simulink model "testModel"  (R2024b)
settings: Solver=ode8  StartTime=0.0  StopTime=10.0  FixedStep=0.025  RelTol=1e-3
values from neighbouring files (symbols this model uses):
  I = diag(Iv)    [InitTest.m]
  invI = inv(I)    [InitTest.m]
  R = 42000000    [InitTest.m]
  w0 = [1e-6; 1e-6; orb.n]    [InitTest.m]
undefined symbols (not defined in the file or in its folder): env, flag, IC, orb
libraries: matrix_library x2
settings Model: SimulationMode=accelerator  Creator=elisa  LastModifiedBy=filippocamaleonte

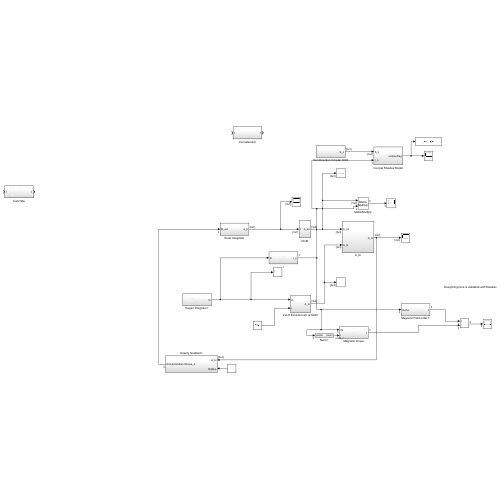
[thumbnail: Simulink's stored preview of the top-level diagram]
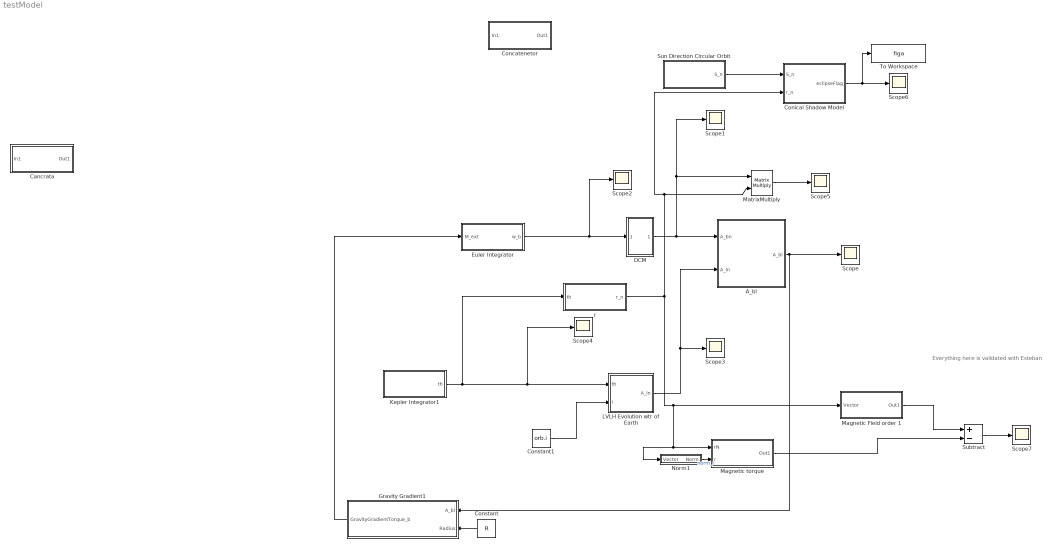
== system testModel ==
  note: Everything here is validated with Esteban
  A_bl : Subsystem
  Cancrata : Subsystem
  Concatenetor : Subsystem
  Conical Shadow Model : Subsystem
  Constant : Constant  Value=R
  Constant1 : Constant  Value=orb.i
  DCM : Subsystem
  Euler Integrator : Subsystem
  Gravity Gradient1 : Subsystem
  Kepler Integrator1 : Subsystem
  LVLH Evolution wtr of Earth : Subsystem
  Magnetic Field order 1 : Subsystem
  Magnetic torque : Subsystem
  MatrixMultiply : Product  Multiplication=Matrix(*)
  Norm1 : Subsystem
  Scope{,1..7} (8 alike) : Scope
  Subtract : Sum  Inputs=+-
  Sun Direction Circular Orbit : Subsystem
  To Workspace : ToWorkspace  VariableName=figa  SampleTime=-1
  r : Subsystem
  wires:
  Euler Integrator/1(w_b) -> Scope2/1, DCM/1(In1)
  DCM/1(A_bn) -> Scope1/1, MatrixMultiply/1, A_bl/1(A_bn)
  LVLH Evolution wtr of Earth/1(A_ln) -> Scope3/1, A_bl/2(A_ln)
  A_bl/1(A_bl) -> Scope/1, Gravity Gradient1/1(A_bl)
  Constant/1 -> Gravity Gradient1/2(Radius)
  Gravity Gradient1/1(GravityGradientTorque_b) -> Euler Integrator/1(M_ext)
  Kepler Integrator1/1(th) -> r/1(th), LVLH Evolution wtr of Earth/1(th), Scope4/1
  Constant1/1 -> LVLH Evolution wtr of Earth/2(i)
  MatrixMultiply/1 -> Scope5/1
  Sun Direction Circular Orbit/1(S_n) -> Conical Shadow Model/1(S_n)
  Conical Shadow Model/1(eclipseFlag) -> To Workspace/1, Scope6/1
  Norm1/1(Norm) -> Magnetic torque/2(r)  "norm_r"
  r/1(r_n) -> Norm1/1(Vector), Magnetic torque/1(rN), Magnetic Field order 1/1(Vector), MatrixMultiply/2, Conical Shadow Model/2(r_n)
  Subtract/1 -> Scope7/1
  Magnetic Field order 1/1(Out1) -> Subtract/1
  Magnetic torque/1(Out1) -> Subtract/2

== system testModel/A_bl ==
  A_bn : Inport
  A_ln : Inport  Port=2
  Matrix Multiply : Product  Multiplication=Matrix(*)
  Transpose : Math  Operator=transpose
  A_bl : Outport
  wires:
  Transpose/1 -> Matrix Multiply/2
  A_ln/1 -> Transpose/1
  Matrix Multiply/1 -> A_bl/1
  A_bn/1 -> Matrix Multiply/1

== system testModel/Cancrata ==
  In1 : Inport
  K_nm : Subsystem
  P_0 : Subsystem
  Pnn : Subsystem
  dPnn : Subsystem
  Out1 : Outport
  wires:
  In1/1 -> Out1/1

== system testModel/Concatenetor ==
  In1 : Inport
  Matrix Concatenate : Concatenate  NumInputs=3  Mode=Multidimensional array  ConcatenateDimension=2
  Out1 : Outport
  wires:
  Matrix Concatenate/1 -> Out1/1
  In1/1 -> Matrix Concatenate/3, Matrix Concatenate/1, Matrix Concatenate/2

== system testModel/Conical Shadow Model ==
  note: Output Interface
  note: Input Interface
  note: Model is cylindrical shadow, formula was taken by Crassidis
  S_n : Inport
  r_n : Inport  Port=2
  Dot Product : DotProduct  OutDataTypeStr=Inherit: Inherit via internal rule
  Earth's Radius : Constant  Value=env.Earth.R
  Eclipse (1) : Subsystem  TreatAsAtomicUnit=on
  Gain : Gain  Gain=-1
  If : If  NumInputs=2  IfExpression=u1 < u2
  Merge : Merge
  Norm : Subsystem
  NotEclipse (0) : Subsystem  TreatAsAtomicUnit=on
  Sqrt : Sqrt
  Square : Math  Operator=square
  Square1 : Math  Operator=square
  Subtract : Sum  Inputs=+-
  eclipseFlag : Outport
  wires:
  r_n/1 -> Dot Product/2, Norm/1(Vector)  "r_n"
  S_n/1 -> Dot Product/1  "S_n"
  Norm/1(Norm) -> Square1/1  "norm_r"
  If/1 -> Eclipse (1)/Action
  If/2 -> NotEclipse (0)/Action
  Merge/1 -> eclipseFlag/1
  Eclipse (1)/1(One) -> Merge/1
  NotEclipse (0)/1(Zero) -> Merge/2
  Dot Product/1 -> If/1
  Gain/1 -> If/2
  Sqrt/1 -> Gain/1
  Subtract/1 -> Sqrt/1
  Square/1 -> Subtract/2
  Square1/1 -> Subtract/1
  Earth's Radius/1 -> Square/1  "earth_R"

== system testModel/DCM ==
  In1 : Inport
  A312 : Subsystem
  Constant3 : Constant  Value=IC.angles
  Gain : Gain  Gain=-1
  Integrator1 : Integrator  InitialConditionSource=external
  Product1 : Product  Multiplication=Matrix(*)
  Subsystem : Subsystem
  Subsystem1 : Subsystem
  Subsystem2 : Subsystem
  w^ : Subsystem
  A_bn : Outport
  wires:
  w^/1(Out1) -> Gain/1
  Gain/1 -> Product1/1
  In1/1 -> w^/1(In1)
  Product1/1 -> Integrator1/1
  Constant3/1 -> A312/1(In1)
  Integrator1/1 -> Subsystem/1(In1)
  Subsystem/1(Out1) -> Subsystem1/1(In1)
  A312/1(Out1) -> Integrator1/2
  Subsystem1/1(Out1) -> Subsystem2/1(In1)
  Subsystem2/1(Out1) -> Product1/2, A_bn/1

== system testModel/Euler Integrator ==
  M_ext : Inport
  Constant : Constant  Value=I
  Constant1 : Constant  Value=w0  VectorParams1D=off
  Constant2 : Constant  Value=invI
  Cross Product : matrix_library/Cross Product
  Divide : Product  Inputs=**  Multiplication=Matrix(*)
  Integrator : Integrator  InitialConditionSource=external
  Product : Product  Multiplication=Matrix(*)
  Sum : Sum  Inputs=|++
  w_b : Outport
  wires:
  Product/1 -> Cross Product/1
  Divide/1 -> Integrator/1
  Constant/1 -> Product/1
  Constant2/1 -> Divide/1
  Integrator/1 -> Product/2, Cross Product/2, w_b/1
  Constant1/1 -> Integrator/2
  Cross Product/1 -> Sum/1
  Sum/1 -> Divide/2
  M_ext/1 -> Sum/2

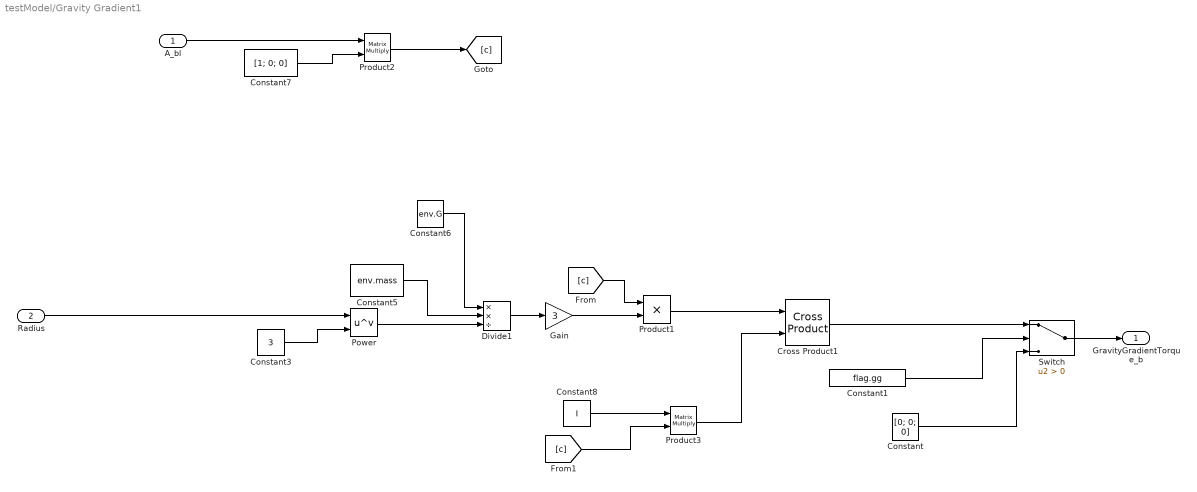
== system testModel/Gravity Gradient1 ==
  A_bl : Inport
  Radius : Inport  Port=2
  Constant : Constant  Value=[0; 0; 0]
  Constant1 : Constant  Value=flag.gg
  Constant3 : Constant  Value=3
  Constant5 : Constant  Value=env.mass
  Constant6 : Constant  Value=env.G
  Constant7 : Constant  Value=[1; 0; 0]
  Constant8 : Constant  Value=I
  Cross Product1 : matrix_library/Cross Product
  Divide1 : Product  Inputs=**/
  Gain : Gain  Gain=3
  Power : Math  Operator=pow
  Product1 : Product
  Product2 : Product  Multiplication=Matrix(*)
  Product3 : Product  Multiplication=Matrix(*)
  Switch : Switch  Criteria=u2 > Threshold  SaturateOnIntegerOverflow=off  InputSameDT=off
  GravityGradientTorque_b : Outport
  wires:
  A_bl/1 -> Product2/1
  Product3/1 -> Cross Product1/2
  Product2/1 -> [c]
  Constant8/1 -> Product3/1
  Product1/1 -> Cross Product1/1
  [c] -> Product1/1
  [c] -> Product3/2
  Constant6/1 -> Divide1/1
  Constant5/1 -> Divide1/2
  Radius/1 -> Power/1
  Constant7/1 -> Product2/2
  Constant3/1 -> Power/2
  Power/1 -> Divide1/3
  Divide1/1 -> Gain/1
  Gain/1 -> Product1/2
  Constant/1 -> Switch/3
  Switch/1 -> GravityGradientTorque_b/1
  Cross Product1/1 -> Switch/1
  Constant1/1 -> Switch/2

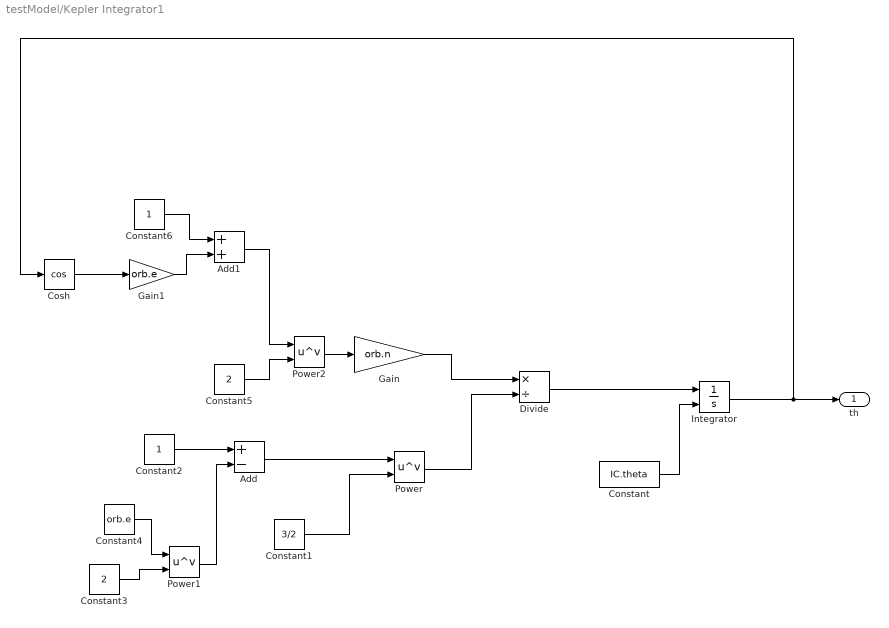
== system testModel/Kepler Integrator1 ==
  Add : Sum  Inputs=+-
  Add1 : Sum
  Constant : Constant  Value=IC.theta
  Constant1 : Constant  Value=3/2
  Constant2 : Constant
  Constant3 : Constant  Value=2
  Constant4 : Constant  Value=orb.e
  Constant5 : Constant  Value=2
  Constant6 : Constant
  Cosh : Trigonometry  Operator=cos
  Divide : Product  Inputs=*/
  Gain : Gain  Gain=orb.n
  Gain1 : Gain  Gain=orb.e
  Integrator : Integrator  InitialConditionSource=external  WrapState=on  WrappedStateUpperValue=2*pi  WrappedStateLowerValue=0
  Power : Math  Operator=pow
  Power1 : Math  Operator=pow
  Power2 : Math  Operator=pow
  th : Outport
  wires:
  Constant/1 -> Integrator/2
  Integrator/1 -> Cosh/1, th/1
  Divide/1 -> Integrator/1
  Power/1 -> Divide/2
  Constant1/1 -> Power/2
  Constant2/1 -> Add/1
  Add/1 -> Power/1
  Power1/1 -> Add/2
  Constant3/1 -> Power1/2
  Constant4/1 -> Power1/1
  Gain/1 -> Divide/1
  Power2/1 -> Gain/1
  Constant5/1 -> Power2/2
  Add1/1 -> Power2/1
  Constant6/1 -> Add1/1
  Gain1/1 -> Add1/2
  Cosh/1 -> Gain1/1

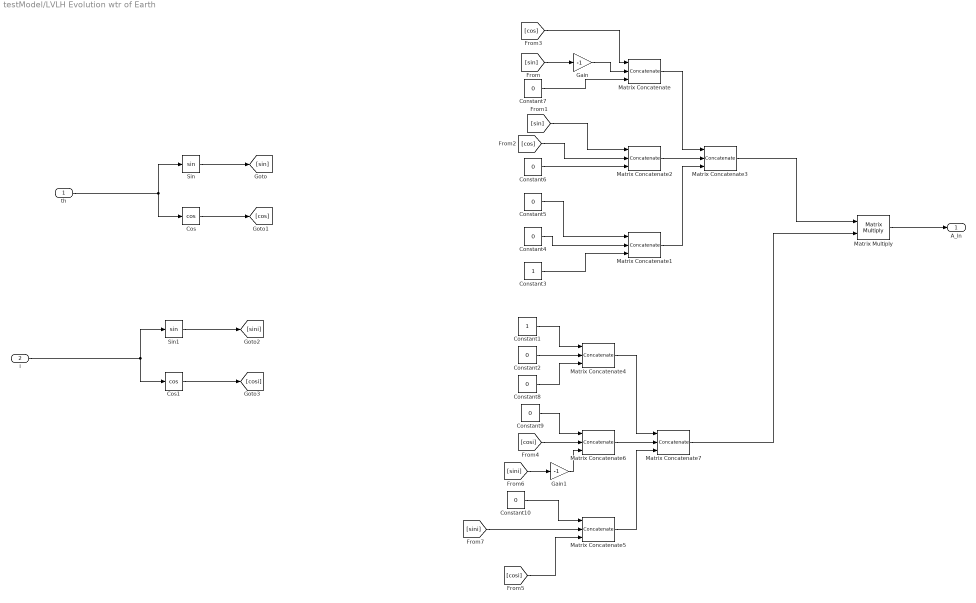
== system testModel/LVLH Evolution wtr of Earth ==
  th : Inport
  i : Inport  Port=2
  Constant1 : Constant
  Constant{2,4..10} (8 alike) : Constant  Value=0
  Constant3 : Constant
  Cos : Trigonometry  Operator=cos
  Cos1 : Trigonometry  Operator=cos
  Gain : Gain  Gain=-1
  Gain1 : Gain  Gain=-1
  Matrix Concatenate{,1..2,4..6} (6 alike) : Concatenate  NumInputs=3  Mode=Multidimensional array
  Matrix Concatenate3 : Concatenate  NumInputs=3  Mode=Multidimensional array  ConcatenateDimension=2
  Matrix Concatenate7 : Concatenate  NumInputs=3  Mode=Multidimensional array  ConcatenateDimension=2
  Matrix Multiply : Product  Multiplication=Matrix(*)
  Sin : Trigonometry
  Sin1 : Trigonometry
  A_ln : Outport
  wires:
  Cos/1 -> [cos]
  Matrix Concatenate1/1 -> Matrix Concatenate3/3
  th/1 -> Cos/1, Sin/1
  Matrix Concatenate/1 -> Matrix Concatenate3/1
  Constant5/1 -> Matrix Concatenate1/1
  Constant3/1 -> Matrix Concatenate1/3
  [cos] -> Matrix Concatenate/1
  Sin/1 -> [sin]
  Constant6/1 -> Matrix Concatenate2/3
  Constant7/1 -> Matrix Concatenate/3
  Constant4/1 -> Matrix Concatenate1/2
  Matrix Concatenate2/1 -> Matrix Concatenate3/2
  [cos] -> Matrix Concatenate2/2
  [sin] -> Matrix Concatenate2/1
  Gain/1 -> Matrix Concatenate/2
  [sin] -> Gain/1
  Cos1/1 -> [cosi]
  Sin1/1 -> [sini]
  i/1 -> Cos1/1, Sin1/1
  Matrix Multiply/1 -> A_ln/1
  Matrix Concatenate3/1 -> Matrix Multiply/1
  Matrix Concatenate7/1 -> Matrix Multiply/2
  Matrix Concatenate6/1 -> Matrix Concatenate7/2
  Matrix Concatenate5/1 -> Matrix Concatenate7/3
  Matrix Concatenate4/1 -> Matrix Concatenate7/1
  Constant1/1 -> Matrix Concatenate4/1
  Constant2/1 -> Matrix Concatenate4/2
  Constant8/1 -> Matrix Concatenate4/3
  Constant9/1 -> Matrix Concatenate6/1
  Constant10/1 -> Matrix Concatenate5/1
  [cosi] -> Matrix Concatenate5/3
  [cosi] -> Matrix Concatenate6/2
  [sini] -> Matrix Concatenate5/2
  [sini] -> Gain1/1
  Gain1/1 -> Matrix Concatenate6/3

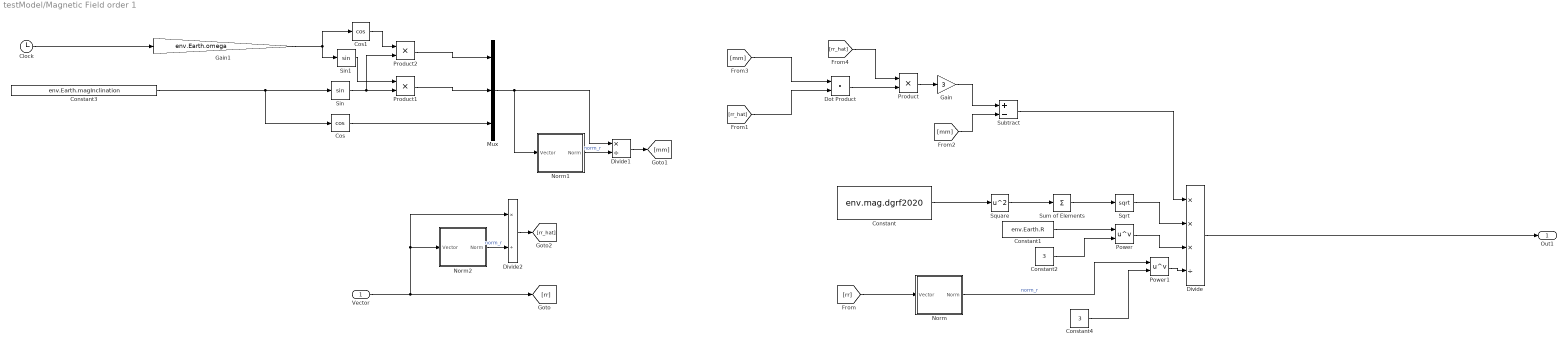
== system testModel/Magnetic Field order 1 ==
  Vector : Inport
  Clock : Clock
  Constant : Constant  Value=env.mag.dgrf2020
  Constant1 : Constant  Value=env.Earth.R
  Constant2 : Constant  Value=3
  Constant3 : Constant  Value=env.Earth.magInclination
  Constant4 : Constant  Value=3
  Cos : Trigonometry  Operator=cos
  Cos1 : Trigonometry  Operator=cos
  Divide : Product  Inputs=***/
  Divide1 : Product  Inputs=*/
  Divide2 : Product  Inputs=*/
  Dot Product : DotProduct  OutDataTypeStr=Inherit: Inherit via internal rule
  Gain : Gain  Gain=3
  Gain1 : Gain  Gain=env.Earth.omega
  Mux : Mux  Inputs=3
  Norm : Subsystem
  Norm1 : Subsystem
  Norm2 : Subsystem
  Power : Math  Operator=pow
  Power1 : Math  Operator=pow
  Product : Product
  Product1 : Product
  Product2 : Product
  Sin : Trigonometry
  Sin1 : Trigonometry
  Sqrt : Sqrt
  Square : Math  Operator=square
  Subtract : Sum  Inputs=+-
  Sum of Elements : Sum  Inputs=+
  Out1 : Outport
  wires:
  Constant/1 -> Square/1
  Square/1 -> Sum of Elements/1
  Sum of Elements/1 -> Sqrt/1
  Constant1/1 -> Power/1
  Constant2/1 -> Power/2
  Sqrt/1 -> Divide/2
  Power/1 -> Divide/3
  Constant4/1 -> Power1/2
  Power1/1 -> Divide/4
  Norm/1(Norm) -> Power1/1  "norm_r"
  Vector/1 -> Norm2/1(Vector), Divide2/1, [rr]
  [rr] -> Norm/1(Vector)
  [rr_hat] -> Dot Product/2
  Subtract/1 -> Divide/1
  [mm] -> Subtract/2
  Dot Product/1 -> Product/2
  Product/1 -> Gain/1
  Gain/1 -> Subtract/1
  [rr_hat] -> Product/1
  [mm] -> Dot Product/1
  Mux/1 -> Norm1/1(Vector), Divide1/1
  Cos/1 -> Mux/3
  Constant3/1 -> Sin/1, Cos/1
  Clock/1 -> Gain1/1
  Sin/1 -> Product2/2, Product1/2
  Product1/1 -> Mux/2
  Product2/1 -> Mux/1
  Cos1/1 -> Product2/1
  Gain1/1 -> Cos1/1, Sin1/1
  Sin1/1 -> Product1/1
  Divide/1 -> Out1/1
  Norm1/1(Norm) -> Divide1/2  "norm_r"
  Divide1/1 -> [mm]
  Norm2/1(Norm) -> Divide2/2  "norm_r"
  Divide2/1 -> [rr_hat]

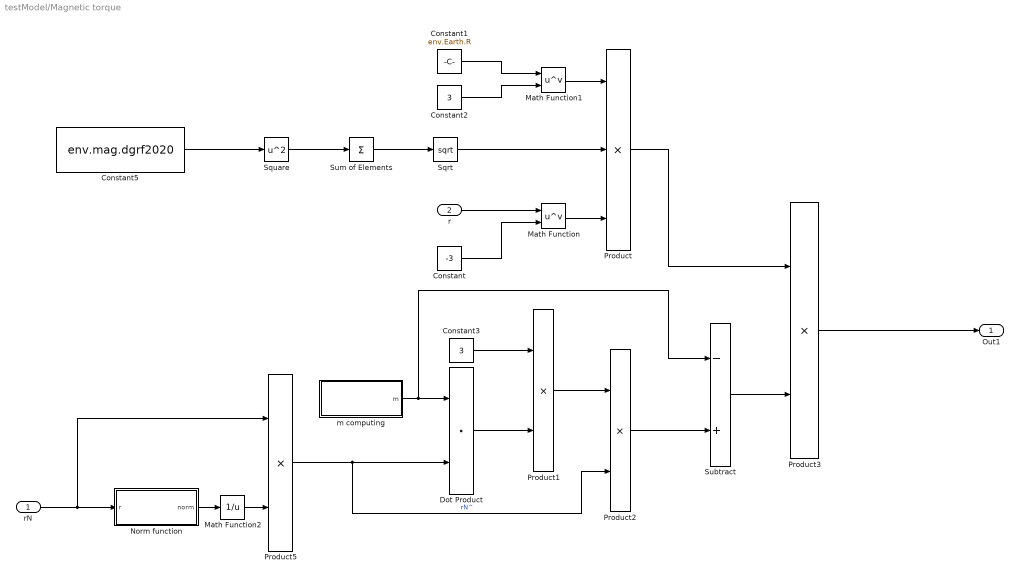
== system testModel/Magnetic torque ==
  rN : Inport
  r : Inport  Port=2
  Constant : Constant  Value=-3
  Constant1 : Constant  Value=env.Earth.R
  Constant2 : Constant  Value=3
  Constant3 : Constant  Value=3
  Constant5 : Constant  Value=env.mag.dgrf2020
  Dot Product : DotProduct  OutDataTypeStr=Inherit: Inherit via internal rule
  Math Function : Math  Operator=pow
  Math Function1 : Math  Operator=pow
  Math Function2 : Math  Operator=reciprocal
  Norm function : Subsystem
  Product : Product  Inputs=3
  Product{1..3,5} (4 alike) : Product
  Sqrt : Sqrt
  Square : Math  Operator=square
  Subtract : Sum  Inputs=-+
  Sum of Elements : Sum  Inputs=+
  m computing : Subsystem
  Out1 : Outport
  wires:
  Sqrt/1 -> Product/2
  Constant3/1 -> Product1/1
  Math Function1/1 -> Product/1
  Product/1 -> Product3/1
  Product1/1 -> Product2/1
  Math Function2/1 -> Product5/2
  Constant/1 -> Math Function/2
  Dot Product/1 -> Product1/2
  Product5/1 -> Dot Product/2, Product2/2  "rN^"
  Constant1/1 -> Math Function1/1
  Constant2/1 -> Math Function1/2
  Product2/1 -> Subtract/2
  rN/1 -> Product5/1, Norm function/1(r)
  Norm function/1(norm) -> Math Function2/1
  r/1 -> Math Function/1
  m computing/1(m) -> Dot Product/1, Subtract/1
  Math Function/1 -> Product/3
  Subtract/1 -> Product3/2
  Sum of Elements/1 -> Sqrt/1
  Constant5/1 -> Square/1
  Square/1 -> Sum of Elements/1
  Product3/1 -> Out1/1

== system testModel/Norm1 ==
  Vector : Inport
  Add : Sum  Inputs=+++
  Demux : Demux  Outputs=3
  Sqrt : Sqrt
  Square : Math  Operator=square
  Square1 : Math  Operator=square
  Square2 : Math  Operator=square
  Norm : Outport
  wires:
  Square/1 -> Add/1
  Add/1 -> Sqrt/1
  Demux/3 -> Square1/1
  Square2/1 -> Add/2
  Square1/1 -> Add/3
  Demux/1 -> Square/1
  Demux/2 -> Square2/1
  Vector/1 -> Demux/1
  Sqrt/1 -> Norm/1

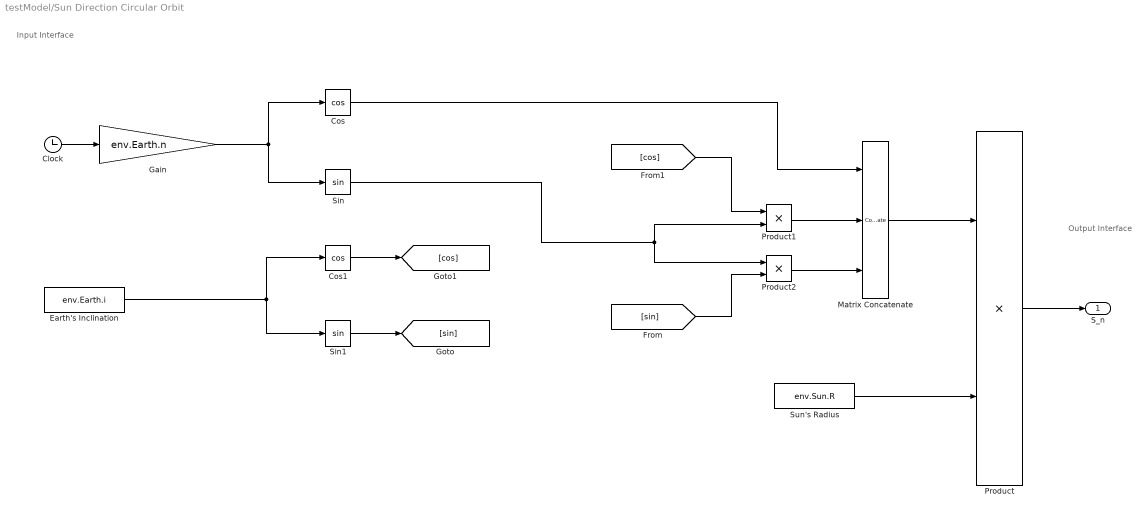
== system testModel/Sun Direction Circular Orbit ==
  note: Input Interface
  note: Output Interface
  Clock : Clock
  Cos : Trigonometry  Operator=cos
  Cos1 : Trigonometry  Operator=cos
  Earth's Inclination : Constant  Value=env.Earth.i
  Gain : Gain  Gain=env.Earth.n
  Matrix Concatenate : Concatenate  NumInputs=3  Mode=Multidimensional array
  Product : Product
  Product1 : Product
  Product2 : Product
  Sin : Trigonometry
  Sin1 : Trigonometry
  Sun's Radius : Constant  Value=env.Sun.R
  S_n : Outport
  wires:
  Clock/1 -> Gain/1
  Gain/1 -> Sin/1, Cos/1
  Product/1 -> S_n/1
  Sun's Radius/1 -> Product/2
  Matrix Concatenate/1 -> Product/1
  Earth's Inclination/1 -> Sin1/1, Cos1/1
  Cos1/1 -> [cos]
  Sin1/1 -> [sin]
  Cos/1 -> Matrix Concatenate/1
  Product1/1 -> Matrix Concatenate/2
  Product2/1 -> Matrix Concatenate/3
  [sin] -> Product2/2
  [cos] -> Product1/1
  Sin/1 -> Product1/2, Product2/1

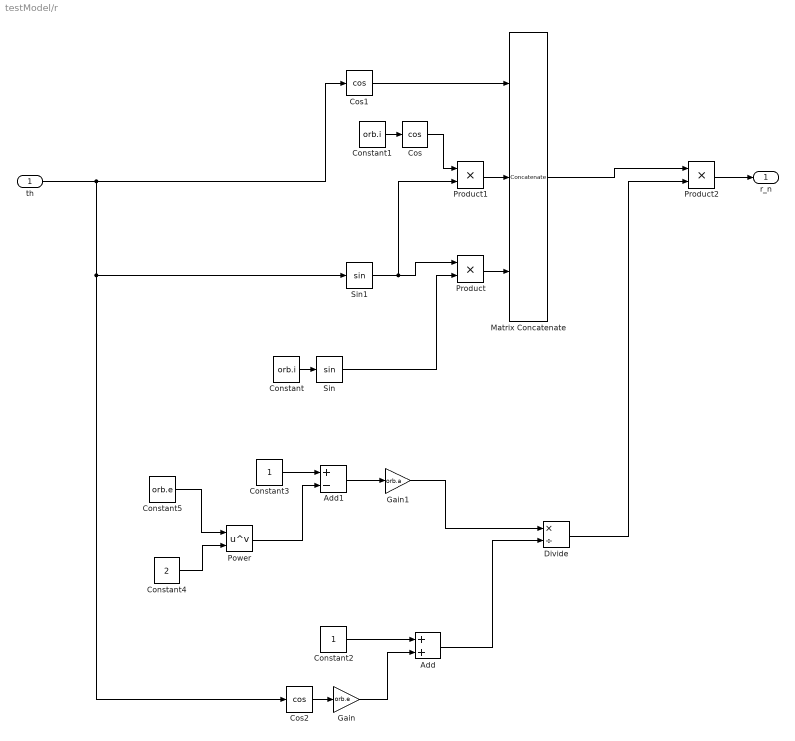
== system testModel/r ==
  th : Inport
  Add : Sum
  Add1 : Sum  Inputs=+-
  Constant : Constant  Value=orb.i
  Constant1 : Constant  Value=orb.i
  Constant2 : Constant
  Constant3 : Constant
  Constant4 : Constant  Value=2
  Constant5 : Constant  Value=orb.e
  Cos : Trigonometry  Operator=cos
  Cos1 : Trigonometry  Operator=cos
  Cos2 : Trigonometry  Operator=cos
  Divide : Product  Inputs=*/
  Gain : Gain  Gain=orb.e
  Gain1 : Gain  Gain=orb.a
  Matrix Concatenate : Concatenate  NumInputs=3  Mode=Multidimensional array
  Power : Math  Operator=pow
  Product : Product
  Product1 : Product
  Product2 : Product
  Sin : Trigonometry
  Sin1 : Trigonometry
  r_n : Outport
  wires:
  Constant/1 -> Sin/1
  Cos1/1 -> Matrix Concatenate/1
  th/1 -> Sin1/1, Cos2/1, Cos1/1
  Product1/1 -> Matrix Concatenate/2
  Product/1 -> Matrix Concatenate/3
  Sin1/1 -> Product1/2, Product/1
  Sin/1 -> Product/2
  Constant1/1 -> Cos/1
  Cos/1 -> Product1/1
  Product2/1 -> r_n/1
  Matrix Concatenate/1 -> Product2/1
  Divide/1 -> Product2/2
  Constant2/1 -> Add/1
  Add/1 -> Divide/2
  Cos2/1 -> Gain/1
  Gain/1 -> Add/2
  Constant3/1 -> Add1/1
  Power/1 -> Add1/2
  Constant4/1 -> Power/2
  Constant5/1 -> Power/1
  Add1/1 -> Gain1/1
  Gain1/1 -> Divide/1

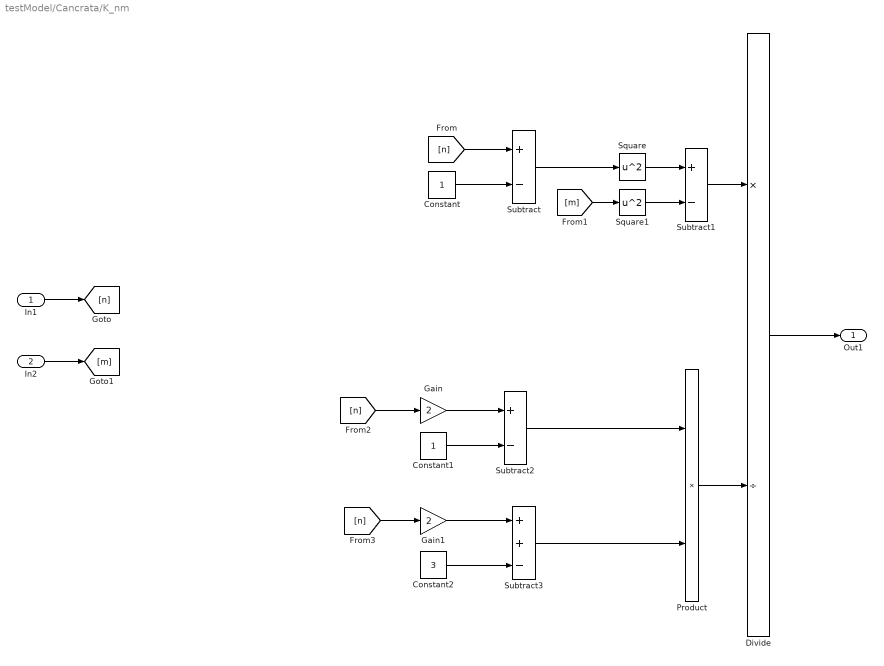
== system testModel/Cancrata/K_nm ==
  In1 : Inport
  In2 : Inport  Port=2
  Constant : Constant
  Constant1 : Constant
  Constant2 : Constant  Value=3
  Divide : Product  Inputs=*/
  Gain : Gain  Gain=2
  Gain1 : Gain  Gain=2
  Product : Product
  Square : Math  Operator=square
  Square1 : Math  Operator=square
  Subtract : Sum  Inputs=+-
  Subtract1 : Sum  Inputs=+-
  Subtract2 : Sum  Inputs=+-
  Subtract3 : Sum  Inputs=++-
  Out1 : Outport
  wires:
  In1/1 -> [n]
  In2/1 -> [m]
  [n] -> Subtract/1
  Constant/1 -> Subtract/2
  Subtract/1 -> Square/1
  Square/1 -> Subtract1/1
  [m] -> Square1/1
  Square1/1 -> Subtract1/2
  Subtract1/1 -> Divide/1
  Divide/1 -> Out1/1
  Product/1 -> Divide/2
  [n] -> Gain/1
  Constant1/1 -> Subtract2/2
  Gain/1 -> Subtract2/1
  Subtract2/1 -> Product/1
  Subtract3/1 -> Product/2
  Constant2/1 -> Subtract3/3
  Gain1/1 -> Subtract3/1
  [n] -> Gain1/1

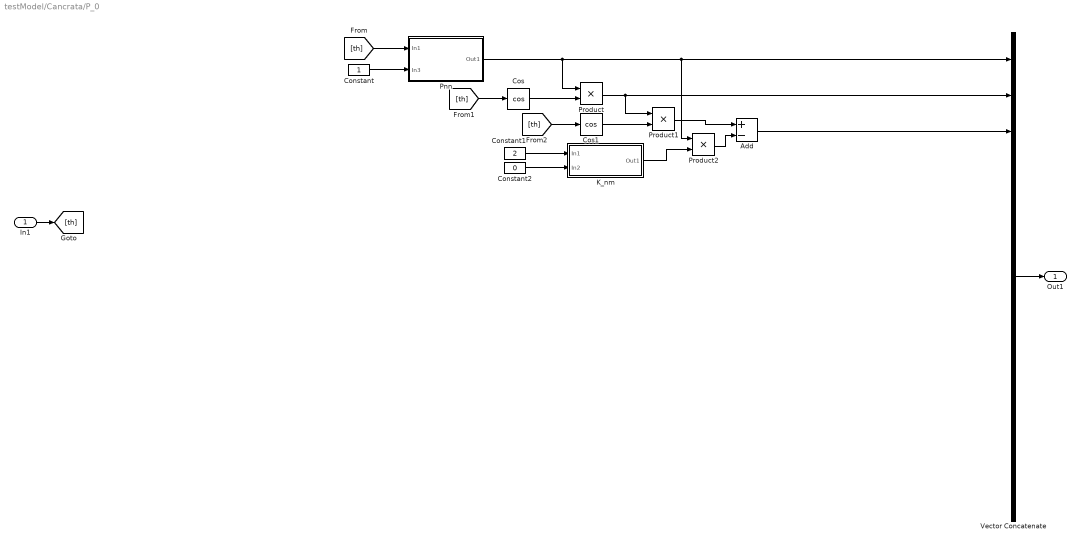
== system testModel/Cancrata/P_0 ==
  In1 : Inport
  Add : Sum  Inputs=+-
  Constant : Constant
  Constant1 : Constant  Value=2
  Constant2 : Constant  Value=0
  Cos : Trigonometry  Operator=cos
  Cos1 : Trigonometry  Operator=cos
  K_nm : Subsystem
  Pnn : Subsystem
  Product : Product
  Product1 : Product
  Product2 : Product
  Vector Concatenate : Concatenate  NumInputs=13
  Out1 : Outport
  wires:
  Vector Concatenate/1 -> Out1/1
  Constant/1 -> Pnn/2(In3)
  In1/1 -> [th]
  [th] -> Pnn/1(In1)
  Pnn/1(Out1) -> Product2/1, Vector Concatenate/1, Product/1
  Constant2/1 -> K_nm/2(In2)
  Constant1/1 -> K_nm/1(In1)
  [th] -> Cos/1
  Cos/1 -> Product/2
  Product/1 -> Product1/1, Vector Concatenate/2
  Cos1/1 -> Product1/2
  [th] -> Cos1/1
  Add/1 -> Vector Concatenate/3
  Product1/1 -> Add/1
  K_nm/1(Out1) -> Product2/2
  Product2/1 -> Add/2

== system testModel/Cancrata/Pnn ==
  In1 : Inport
  In3 : Inport  Port=2
  Power : Math  Operator=pow
  Sin : Trigonometry
  Out1 : Outport
  wires:
  In3/1 -> Sin/1
  In1/1 -> Power/2
  Sin/1 -> Power/1
  Power/1 -> Out1/1

== system testModel/Cancrata/dPnn ==
  In1 : Inport
  In2 : Inport  Port=2
  Constant : Constant
  Cos : Trigonometry  Operator=cos
  Power : Math  Operator=pow
  Product : Product  Inputs=3
  Sin : Trigonometry
  Subtract : Sum  Inputs=+-
  Out1 : Outport
  wires:
  In2/1 -> Cos/1, Sin/1
  Sin/1 -> Power/1
  In1/1 -> Product/3, Subtract/1
  Constant/1 -> Subtract/2
  Subtract/1 -> Power/2
  Product/1 -> Out1/1
  Cos/1 -> Product/1
  Power/1 -> Product/2

== system testModel/Conical Shadow Model/Eclipse (1) ==
  Action Port : ActionPort  ActionPortLabel=if(u1 < u2)
  Constant : Constant
  One : Outport
  wires:
  Constant/1 -> One/1

== system testModel/Conical Shadow Model/Norm ==
  Vector : Inport
  Add : Sum  Inputs=+++
  Demux : Demux  Outputs=3
  Sqrt : Sqrt
  Square : Math  Operator=square
  Square1 : Math  Operator=square
  Square2 : Math  Operator=square
  Norm : Outport
  wires:
  Square/1 -> Add/1
  Add/1 -> Sqrt/1
  Demux/3 -> Square1/1
  Square2/1 -> Add/2
  Square1/1 -> Add/3
  Demux/1 -> Square/1
  Demux/2 -> Square2/1
  Vector/1 -> Demux/1
  Sqrt/1 -> Norm/1

== system testModel/Conical Shadow Model/NotEclipse (0) ==
  Action Port : ActionPort  ActionPortLabel=else
  Constant : Constant  Value=0
  Zero : Outport
  wires:
  Constant/1 -> Zero/1

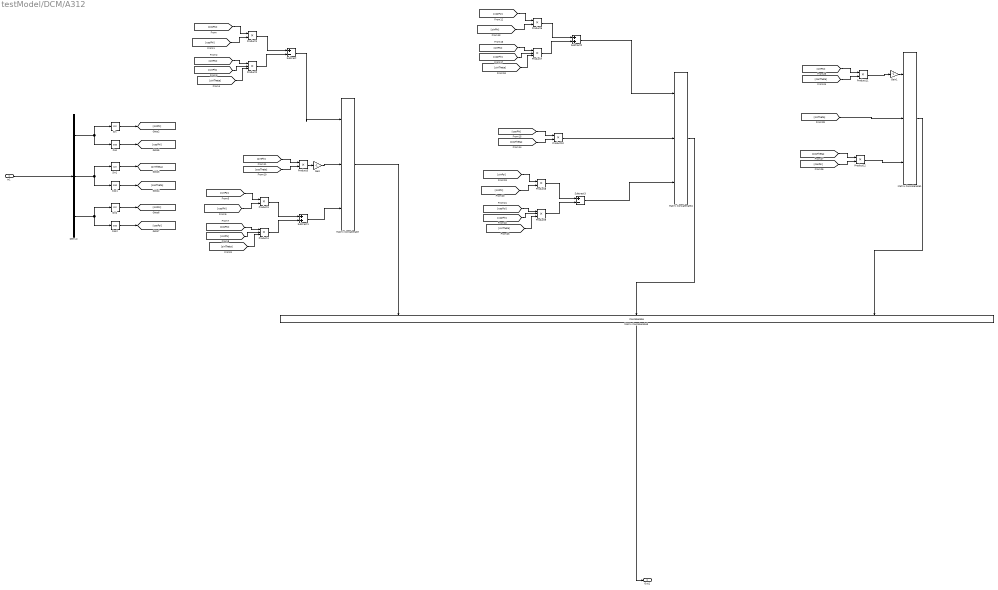
== system testModel/DCM/A312 ==
  In1 : Inport
  Cos : Trigonometry  Operator=cos
  Cos1 : Trigonometry  Operator=cos
  Cos2 : Trigonometry  Operator=cos
  Demux : Demux  Outputs=3
  Gain : Gain  Gain=-1
  Gain1 : Gain  Gain=-1
  Matrix Concatenate : Concatenate  NumInputs=3  Mode=Multidimensional array
  Matrix Concatenate1 : Concatenate  NumInputs=3  Mode=Multidimensional array
  Matrix Concatenate3 : Concatenate  NumInputs=3  Mode=Multidimensional array  ConcatenateDimension=2
  Matrix Concatenate4 : Concatenate  NumInputs=3  Mode=Multidimensional array
  Product{1,3,5..6,8,10..12} (8 alike) : Product
  Product{2,4,7,9} (4 alike) : Product  Inputs=3
  Sin : Trigonometry
  Sin1 : Trigonometry
  Sin2 : Trigonometry
  Subtract : Sum  Inputs=+-
  Subtract1 : Sum
  Subtract2 : Sum
  Subtract3 : Sum  Inputs=+-
  Out1 : Outport
  wires:
  In1/1 -> Demux/1
  [sinTheta] -> Product2/3
  Product7/1 -> Subtract2/2
  [cosTheta] -> Product11/2
  [sinPhi] -> Product8/2
  Sin/1 -> [sinPhi]
  [sinPhi] -> Product2/2
  [cosTheta] -> Product10/2
  [cosPsi] -> Product6/1
  Demux/3 -> Sin2/1, Cos2/1
  Product9/1 -> Subtract3/2
  [sinTheta] -> Matrix Concatenate1/2
  Matrix Concatenate1/1 -> Matrix Concatenate3/3
  [sinPsi] -> Product11/1
  Product2/1 -> Subtract/2
  Subtract2/1 -> Matrix Concatenate4/1
  Matrix Concatenate4/1 -> Matrix Concatenate3/2
  [cosTheta] -> Product12/1
  Cos2/1 -> [cosPsi]
  [sinPsi] -> Product2/1
  [sinPsi] -> Product8/1
  Sin2/1 -> [sinPsi]
  [sinTheta] -> Product7/3
  Subtract/1 -> Matrix Concatenate/1
  [cosPhi] -> Product10/1
  Demux/2 -> Sin1/1, Cos1/1
  [sinTheta] -> Product9/3
  Product8/1 -> Subtract3/1
  [cosPhi] -> Product9/2
  [cosPsi] -> Product9/1
  Product11/1 -> Gain1/1
  Product1/1 -> Subtract/1
  [cosPhi] -> Product1/2
  [cosPsi] -> Product12/2
  [cosPhi] -> Product7/2
  [sinPhi] -> Product6/2
  Product6/1 -> Subtract2/1
  Demux/1 -> Sin/1, Cos/1
  [cosPsi] -> Product1/1
  [sinPsi] -> Product7/1
  Cos1/1 -> [cosTheta]
  Sin1/1 -> [sinTheta]
  Product12/1 -> Matrix Concatenate1/3
  Matrix Concatenate/1 -> Matrix Concatenate3/1
  Cos/1 -> [cosPhi]
  Matrix Concatenate3/1 -> Out1/1
  Gain1/1 -> Matrix Concatenate1/1
  Product10/1 -> Matrix Concatenate4/2
  Subtract3/1 -> Matrix Concatenate4/3
  [cosPsi] -> Product4/1
  Product4/1 -> Subtract1/2
  [cosPhi] -> Product3/2
  Product3/1 -> Subtract1/1
  [sinPsi] -> Product3/1
  [sinPhi] -> Product4/2
  [sinTheta] -> Product4/3
  [sinPhi] -> Product5/1
  [cosTheta] -> Product5/2
  Product5/1 -> Gain/1
  Subtract1/1 -> Matrix Concatenate/3
  Gain/1 -> Matrix Concatenate/2

== system testModel/DCM/Subsystem ==
  In1 : Inport
  Gain1 : Gain  Gain=3/2
  Gain2 : Gain  Gain=1/2
  Product : Product  Inputs=3  Multiplication=Matrix(*)
  Subtract : Sum  Inputs=+-
  Transpose : Math  Operator=transpose
  Out1 : Outport
  wires:
  In1/1 -> Product/3, Product/1, Gain1/1, Transpose/1
  Gain2/1 -> Subtract/2
  Gain1/1 -> Subtract/1
  Product/1 -> Gain2/1
  Transpose/1 -> Product/2
  Subtract/1 -> Out1/1

== system testModel/DCM/Subsystem1 ==
  In1 : Inport
  Gain1 : Gain  Gain=3/2
  Gain2 : Gain  Gain=1/2
  Product : Product  Inputs=3  Multiplication=Matrix(*)
  Subtract : Sum  Inputs=+-
  Transpose : Math  Operator=transpose
  Out1 : Outport
  wires:
  In1/1 -> Product/3, Product/1, Gain1/1, Transpose/1
  Gain2/1 -> Subtract/2
  Gain1/1 -> Subtract/1
  Product/1 -> Gain2/1
  Transpose/1 -> Product/2
  Subtract/1 -> Out1/1

== system testModel/DCM/Subsystem2 ==
  In1 : Inport
  Gain1 : Gain  Gain=3/2
  Gain2 : Gain  Gain=1/2
  Product : Product  Inputs=3  Multiplication=Matrix(*)
  Subtract : Sum  Inputs=+-
  Transpose : Math  Operator=transpose
  Out1 : Outport
  wires:
  In1/1 -> Product/3, Product/1, Gain1/1, Transpose/1
  Gain2/1 -> Subtract/2
  Gain1/1 -> Subtract/1
  Product/1 -> Gain2/1
  Transpose/1 -> Product/2
  Subtract/1 -> Out1/1

== system testModel/DCM/w^ ==
  In1 : Inport
  Constant3 : Constant  Value=0
  Constant4 : Constant  Value=0
  Constant5 : Constant  Value=0
  Demux : Demux  Outputs=3
  Gain : Gain  Gain=-1
  Gain1 : Gain  Gain=-1
  Gain2 : Gain  Gain=-1
  Matrix Concatenate : Concatenate  NumInputs=3  Mode=Multidimensional array  ConcatenateDimension=2
  Matrix Concatenate1 : Concatenate  NumInputs=3  Mode=Multidimensional array
  Matrix Concatenate2 : Concatenate  NumInputs=3  Mode=Multidimensional array
  Matrix Concatenate3 : Concatenate  NumInputs=3  Mode=Multidimensional array
  To Workspace : ToWorkspace  VariableName=merda  SampleTime=-1
  Out1 : Outport
  wires:
  Demux/3 -> Gain1/1, Matrix Concatenate1/2
  Constant4/1 -> Matrix Concatenate1/1
  Matrix Concatenate/1 -> To Workspace/1, Out1/1
  Demux/1 -> Gain2/1, Matrix Concatenate3/3
  Constant5/1 -> Matrix Concatenate3/2
  Matrix Concatenate1/1 -> Matrix Concatenate/1
  Constant3/1 -> Matrix Concatenate2/3
  Matrix Concatenate2/1 -> Matrix Concatenate/3
  Matrix Concatenate3/1 -> Matrix Concatenate/2
  Gain2/1 -> Matrix Concatenate2/2
  Demux/2 -> Matrix Concatenate2/1, Gain/1
  Gain1/1 -> Matrix Concatenate3/1
  Gain/1 -> Matrix Concatenate1/3
  In1/1 -> Demux/1

== system testModel/Magnetic Field order 1/Norm ==
  Vector : Inport
  Add : Sum  Inputs=+++
  Demux : Demux  Outputs=3
  Sqrt : Sqrt
  Square : Math  Operator=square
  Square1 : Math  Operator=square
  Square2 : Math  Operator=square
  Norm : Outport
  wires:
  Square/1 -> Add/1
  Add/1 -> Sqrt/1
  Demux/3 -> Square1/1
  Square2/1 -> Add/2
  Square1/1 -> Add/3
  Demux/1 -> Square/1
  Demux/2 -> Square2/1
  Vector/1 -> Demux/1
  Sqrt/1 -> Norm/1

== system testModel/Magnetic Field order 1/Norm1 ==
  Vector : Inport
  Add : Sum  Inputs=+++
  Demux : Demux  Outputs=3
  Sqrt : Sqrt
  Square : Math  Operator=square
  Square1 : Math  Operator=square
  Square2 : Math  Operator=square
  Norm : Outport
  wires:
  Square/1 -> Add/1
  Add/1 -> Sqrt/1
  Demux/3 -> Square1/1
  Square2/1 -> Add/2
  Square1/1 -> Add/3
  Demux/1 -> Square/1
  Demux/2 -> Square2/1
  Vector/1 -> Demux/1
  Sqrt/1 -> Norm/1

== system testModel/Magnetic Field order 1/Norm2 ==
  Vector : Inport
  Add : Sum  Inputs=+++
  Demux : Demux  Outputs=3
  Sqrt : Sqrt
  Square : Math  Operator=square
  Square1 : Math  Operator=square
  Square2 : Math  Operator=square
  Norm : Outport
  wires:
  Square/1 -> Add/1
  Add/1 -> Sqrt/1
  Demux/3 -> Square1/1
  Square2/1 -> Add/2
  Square1/1 -> Add/3
  Demux/1 -> Square/1
  Demux/2 -> Square2/1
  Vector/1 -> Demux/1
  Sqrt/1 -> Norm/1

== system testModel/Magnetic torque/Norm function ==
  r : Inport
  Add : Sum  Inputs=+++
  Demux : Demux  Outputs=3
  Math Function : Math  Operator=square
  Math Function1 : Math  Operator=square
  Math Function2 : Math  Operator=square
  Sqrt : Sqrt
  norm : Outport
  wires:
  r/1 -> Demux/1
  Math Function2/1 -> Add/2
  Math Function1/1 -> Add/3
  Math Function/1 -> Add/1
  Add/1 -> Sqrt/1
  Sqrt/1 -> norm/1
  Demux/1 -> Math Function/1
  Demux/2 -> Math Function2/1
  Demux/3 -> Math Function1/1

== system testModel/Magnetic torque/m computing ==
  Clock : Clock
  Constant : Constant  Value=env.Earth.omega
  Constant1 : Constant  Value=env.Earth.magInclination
  Mux : Mux  Inputs=3
  Product : Product
  Product4 : Product
  Product5 : Product
  To Workspace : ToWorkspace  VariableName=time  SaveFormat=Timeseries  SampleTime=-1
  Trigonometric Function2 : Trigonometry  Operator=cos
  Trigonometric Function3 : Trigonometry
  Trigonometric Function5 : Trigonometry  Operator=cos
  Trigonometric Function6 : Trigonometry
  m : Outport
  wires:
  Constant1/1 -> Trigonometric Function2/1, Trigonometric Function3/1
  Clock/1 -> Product/2, To Workspace/1
  Mux/1 -> m/1  "m"
  Product/1 -> Trigonometric Function5/1, Trigonometric Function6/1  "wE*t"
  Trigonometric Function5/1 -> Product4/2
  Product4/1 -> Mux/1
  Trigonometric Function6/1 -> Product5/2
  Trigonometric Function3/1 -> Product5/1, Product4/1
  Product5/1 -> Mux/2
  Constant/1 -> Product/1
  Trigonometric Function2/1 -> Mux/3

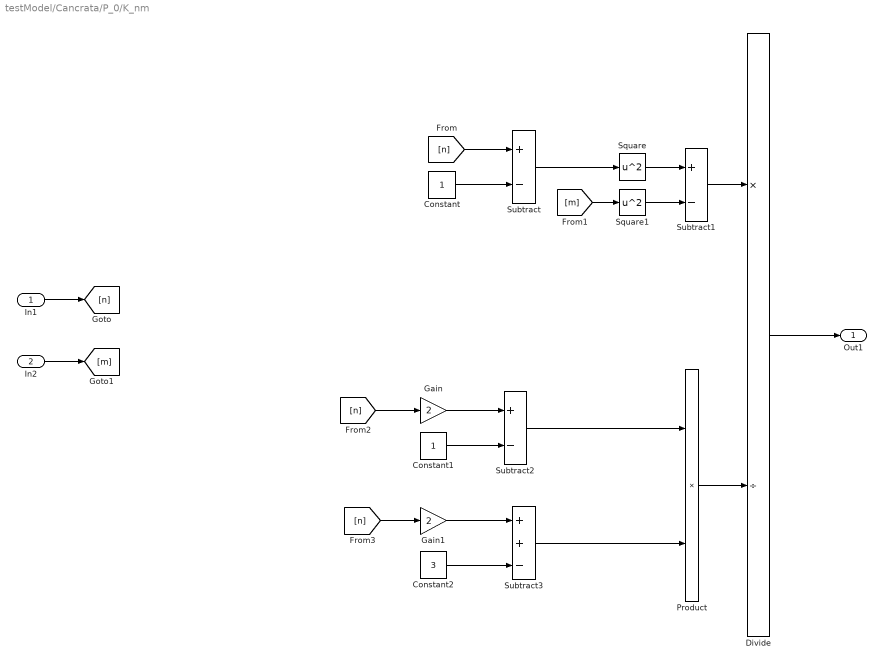
== system testModel/Cancrata/P_0/K_nm ==
  In1 : Inport
  In2 : Inport  Port=2
  Constant : Constant
  Constant1 : Constant
  Constant2 : Constant  Value=3
  Divide : Product  Inputs=*/
  Gain : Gain  Gain=2
  Gain1 : Gain  Gain=2
  Product : Product
  Square : Math  Operator=square
  Square1 : Math  Operator=square
  Subtract : Sum  Inputs=+-
  Subtract1 : Sum  Inputs=+-
  Subtract2 : Sum  Inputs=+-
  Subtract3 : Sum  Inputs=++-
  Out1 : Outport
  wires:
  In1/1 -> [n]
  In2/1 -> [m]
  [n] -> Subtract/1
  Constant/1 -> Subtract/2
  Subtract/1 -> Square/1
  Square/1 -> Subtract1/1
  [m] -> Square1/1
  Square1/1 -> Subtract1/2
  Subtract1/1 -> Divide/1
  Divide/1 -> Out1/1
  Product/1 -> Divide/2
  [n] -> Gain/1
  Constant1/1 -> Subtract2/2
  Gain/1 -> Subtract2/1
  Subtract2/1 -> Product/1
  Subtract3/1 -> Product/2
  Constant2/1 -> Subtract3/3
  Gain1/1 -> Subtract3/1
  [n] -> Gain1/1

== system testModel/Cancrata/P_0/Pnn ==
  In1 : Inport
  In3 : Inport  Port=2
  Power : Math  Operator=pow
  Sin : Trigonometry
  Out1 : Outport
  wires:
  In3/1 -> Sin/1
  In1/1 -> Power/2
  Sin/1 -> Power/1
  Power/1 -> Out1/1
